simulink model "CyberSuspension_MultiBlock"  (R2024b)
settings: Solver=ode4  StartTime=0.0  StopTime=10  FixedStep=0.001  RelTol=1e-3
settings Model: Creator=sange  LastModifiedBy=sange
settings DataIOCC: SaveOutput=off

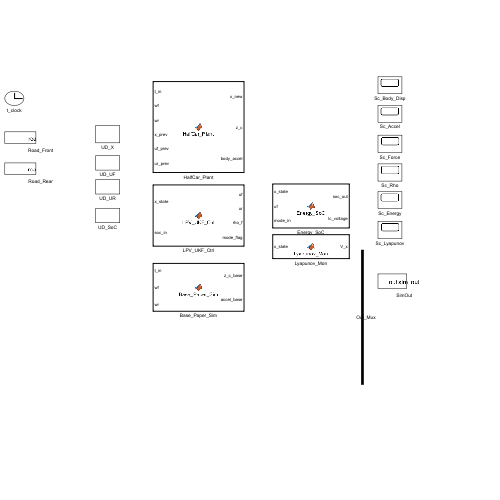
[thumbnail: Simulink's stored preview of the top-level diagram]
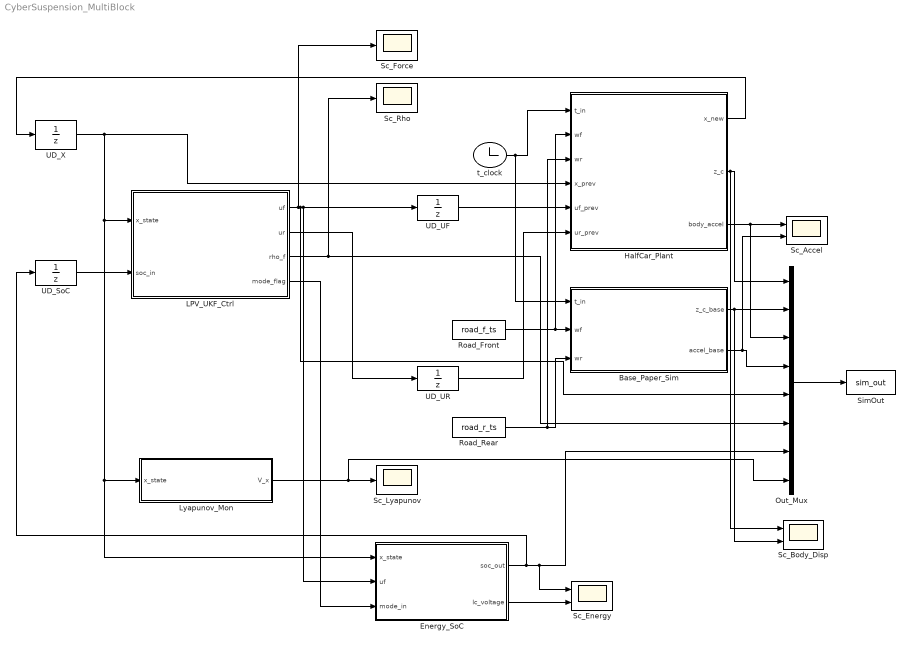
== system CyberSuspension_MultiBlock ==
  Base_Paper_Sim : MATLAB Function  TreatAsAtomicUnit=on
  Energy_SoC : MATLAB Function  TreatAsAtomicUnit=on
  HalfCar_Plant : MATLAB Function  TreatAsAtomicUnit=on
  LPV_UKF_Ctrl : MATLAB Function  TreatAsAtomicUnit=on
  Lyapunov_Mon : MATLAB Function  TreatAsAtomicUnit=on
  Out_Mux : Mux  Inputs=8
  Road_Front : FromWorkspace  VariableName=road_f_ts
  Road_Rear : FromWorkspace  VariableName=road_r_ts
  Sc_Accel : Scope  NumInputPorts=2
  Sc_Body_Disp : Scope  NumInputPorts=2
  Sc_Energy : Scope  NumInputPorts=2
  Sc_Force : Scope
  Sc_Lyapunov : Scope
  Sc_Rho : Scope
  SimOut : ToWorkspace  VariableName=sim_out  SaveFormat=Structure With Time  SampleTime=-1
  UD_SoC : UnitDelay  InitialCondition=0.5  SampleTime=0.001  HasFrameUpgradeWarning=on
  UD_UF : UnitDelay  SampleTime=0.001  HasFrameUpgradeWarning=on
  UD_UR : UnitDelay  SampleTime=0.001  HasFrameUpgradeWarning=on
  UD_X : UnitDelay  InitialCondition=zeros(8,1)  SampleTime=0.001  HasFrameUpgradeWarning=on
  t_clock : Clock
  wires:
  Lyapunov_Mon/1(V_x) -> Sc_Lyapunov/1, Out_Mux/8
  UD_SoC/1 -> LPV_UKF_Ctrl/2(soc_in)
  UD_X/1 -> Energy_SoC/1(x_state), Lyapunov_Mon/1(x_state), LPV_UKF_Ctrl/1(x_state), HalfCar_Plant/4(x_prev)
  LPV_UKF_Ctrl/4(mode_flag) -> Energy_SoC/3(mode_in)
  LPV_UKF_Ctrl/3(rho_f) -> Sc_Rho/1, Out_Mux/6
  Energy_SoC/2(lc_voltage) -> Sc_Energy/2
  LPV_UKF_Ctrl/1(uf) -> UD_UF/1, Energy_SoC/2(uf), Out_Mux/5, Sc_Force/1
  t_clock/1 -> Base_Paper_Sim/1(t_in), HalfCar_Plant/1(t_in)
  LPV_UKF_Ctrl/2(ur) -> UD_UR/1
  UD_UF/1 -> HalfCar_Plant/5(uf_prev)
  Road_Rear/1 -> HalfCar_Plant/3(wr), Base_Paper_Sim/3(wr)
  Road_Front/1 -> HalfCar_Plant/2(wf), Base_Paper_Sim/2(wf)
  UD_UR/1 -> HalfCar_Plant/6(ur_prev)
  Energy_SoC/1(soc_out) -> Out_Mux/7, Sc_Energy/1, UD_SoC/1
  HalfCar_Plant/2(z_c) -> Sc_Body_Disp/1, Out_Mux/1
  HalfCar_Plant/1(x_new) -> UD_X/1
  HalfCar_Plant/3(body_accel) -> Sc_Accel/1, Out_Mux/3
  Base_Paper_Sim/1(z_c_base) -> Sc_Body_Disp/2, Out_Mux/2
  Base_Paper_Sim/2(accel_base) -> Sc_Accel/2, Out_Mux/4
  Out_Mux/1 -> SimOut/1

== matlab function CyberSuspension_MultiBlock/LPV_UKF_Ctrl ==
  data: x_state input; uf output; soc_in input; ur output; rho_f output; mode_flag output
function [uf, ur, rho_f, mode_flag] = LPV_UKF_Ctrl(x_state, soc_in)
% LPV-Adaptive H-inf Controller with UKF Road Estimator + TD3 Heuristic
% Block 2 in the signal chain. Uses x_state from Unit Delay (1ms behind plant).
persistent rho_f_p rdot_filt mets_last mets_first

a=1.10; b=1.50;
C_e=1500; u_max=6000; sig_m=0.10;
w_max=0.05; ema_a=0.05; dt=0.001;
Ks  = [2591.260282 2545.019204 -4409.593492 -22.6009354];
Kr  = [1339.079606 6792.410633 -15288.11257 39.41237591];
Krd = [0 500 0 0];

% Initialise persistent variables (auto-reset at start of each sim run)
if isempty(rho_f_p)
    rho_f_p=0; rdot_filt=0; mets_last=zeros(8,1); mets_first=true;
end

% ---- Step A: METS Network Filter ----
if mets_first
    net=x_state; mets_last=x_state; mets_first=false;
else
    em=x_state-mets_last;
    nx=sqrt(sum(x_state.^2)); ne=sqrt(sum(em.^2));
    if ne>sig_m*nx; mets_last=x_state; net=x_state;
    else;           net=mets_last; end
end

% ---- Step B: UKF Road Estimator (algebraic proxy) ----
rho_f     = min(1, max(0, abs(x_state(1)-a*x_state(2)-x_state(3)) / w_max));
rdot_filt = ema_a*((rho_f-rho_f_p)/dt) + (1-ema_a)*rdot_filt;
rho_dot   = rdot_filt;  rho_f_p = rho_f;

% ---- Step C: TD3 Heuristic Energy Agent ----
if rho_f>0.7 || rho_dot>0.5
    if soc_in<0.02; mf=1; else; mf=0; end   % COMFORT if SoC critical
elseif rho_f>0.3
    if soc_in<0.25; mf=1; else; mf=0; end
else
    mf=1;  % Smooth road — harvest energy (ECO)
end

% ---- Step D: LPV Controller — Polytopic Gain Scheduling ----
zsf=net(1)-a*net(2); zsfd=net(5)-a*net(6); qcf=[zsf-net(3);zsfd;0;net(7)];
zsr=net(1)+b*net(2); zsrd=net(5)+b*net(6); qcr=[zsr-net(4);zsrd;0;net(8)];
ffl = 0.2*u_max;
if mf==1  % ECO: passive regenerative damping
    uf=-C_e*qcf(2);  ur=-C_e*qcr(2);
else       % COMFORT: blended LPV H-inf + feedforward
    Kf = (1-rho_f)*Ks + rho_f*Kr;   % Polytopic interpolation
    uf = (-Kf*qcf) + max(-ffl, min(ffl, -Krd*max(0,rho_dot)*qcf));
    ur = (-Kf*qcr) + max(-ffl, min(ffl, -Krd*max(0,rho_dot)*qcr));
end
uf=max(-u_max,min(u_max,uf));  ur=max(-u_max,min(u_max,ur));
mode_flag = double(mf);
end

== matlab function CyberSuspension_MultiBlock/HalfCar_Plant ==
  data: t_in input; x_new output; wf input; wr input; x_prev input; uf_prev input; ur_prev input; z_c output; body_accel output
function [x_new, z_c, body_accel] = HalfCar_Plant(t_in, wf, wr, x_prev, uf_prev, ur_prev)
% 4-DOF Half-Car Plant with RK4 Integration
% State: [z_c, theta, z_uf, z_ur, z_c_dot, theta_dot, z_uf_dot, z_ur_dot]
% State passed explicitly — no persistent variables needed here.

ms=730.0;  I_phi=1222.0;  a=1.10;  b=1.50;
mu_f=45.0; mu_r=45.0;
ks_f=18000; ks_r=22000; cs_f=1200; cs_r=1200;
kt_f=190000; kt_r=190000;
k_em=15.0; i_d=20.0; p_pole=8; whr=0.30; v_ms=20.00;
smax=0.0800; u_max=6000; k_bs=1.00e+07;
dt = 0.001;

% Runge-Kutta 4 integration (fixed-step, dt=1ms)
k1=hc_ode(t_in,      x_prev,         uf_prev,ur_prev,wf,wr,ms,I_phi,a,b,mu_f,mu_r,ks_f,ks_r,cs_f,cs_r,kt_f,kt_r,k_em,i_d,p_pole,whr,v_ms,smax,k_bs);
k2=hc_ode(t_in+dt/2, x_prev+k1*dt/2, uf_prev,ur_prev,wf,wr,ms,I_phi,a,b,mu_f,mu_r,ks_f,ks_r,cs_f,cs_r,kt_f,kt_r,k_em,i_d,p_pole,whr,v_ms,smax,k_bs);
k3=hc_ode(t_in+dt/2, x_prev+k2*dt/2, uf_prev,ur_prev,wf,wr,ms,I_phi,a,b,mu_f,mu_r,ks_f,ks_r,cs_f,cs_r,kt_f,kt_r,k_em,i_d,p_pole,whr,v_ms,smax,k_bs);
k4=hc_ode(t_in+dt,   x_prev+k3*dt,   uf_prev,ur_prev,wf,wr,ms,I_phi,a,b,mu_f,mu_r,ks_f,ks_r,cs_f,cs_r,kt_f,kt_r,k_em,i_d,p_pole,whr,v_ms,smax,k_bs);
x_new      = x_prev + (dt/6)*(k1 + 2*k2 + 2*k3 + k4);
z_c        = x_new(1);
body_accel = k1(5);
end

function dx = hc_ode(t,x,uf,ur,wf,wr,ms,Ip,a,b,muf,mur,ksf,ksr,csf,csr,ktf,ktr,kem,id,pp,whr,vms,sm,kbs)
    z_c=x(1);th=x(2);zuf=x(3);zur=x(4);zcd=x(5);thd=x(6);zufd=x(7);zurd=x(8);
    zsf=z_c-a*th; zsr=z_c+b*th; zsfd=zcd-a*thd; zsrd=zcd+b*thd;
    dsf=zsf-zuf; dsr=zsr-zur; dtf=zuf-wf; dtr=zur-wr;
    vrf=zsfd-zufd; vrr=zsrd-zurd;
    if dsf> sm; fbf=kbs*(dsf-sm)^3; elseif dsf<-sm; fbf=kbs*(dsf+sm)^3; else; fbf=0; end
    if dsr> sm; fbr=kbs*(dsr-sm)^3; elseif dsr<-sm; fbr=kbs*(dsr+sm)^3; else; fbr=0; end
    fiwm = kem*id*sin(pp*(vms/whr)*t);
    Fsf=ksf*dsf+csf*vrf+fbf-uf; Fsr=ksr*dsr+csr*vrr+fbr-ur;
    dx=[zcd;thd;zufd;zurd; -(Fsf+Fsr)/ms; (a*Fsf-b*Fsr)/Ip; (Fsf-ktf*dtf+fiwm)/muf; (Fsr-ktr*dtr+fiwm)/mur];
end

== matlab function CyberSuspension_MultiBlock/Energy_SoC ==
  data: x_state input; soc_out output; uf input; mode_in input; lc_voltage output
function [soc_out, lc_voltage] = Energy_SoC(x_state, uf, mode_in)
% LC Filter Power Electronics + Regenerative Energy Harvesting
% Tracks battery State-of-Charge and LC filter capacitor voltage.
persistent bat_soc lc_il lc_vc

a=1.10; K_v=50.0; eta_r=0.65; eta_act=0.85;
Lf=0.0100; Cf=0.004700; Rl=10.0; cap_j=50000; dt=0.001;
N_t=10.0; % Lightweight Transformer/Boost step-up ratio

if isempty(bat_soc); bat_soc=0.5; lc_il=0; lc_vc=0; end

% Relative suspension velocity (front corner)
vrf = (x_state(5) - a*x_state(6)) - x_state(7);

if mode_in == 1  % ECO mode: harvest energy via back-EMF
    v_rect = abs(K_v * vrf) * N_t; % Voltage is boosted by transformer
    di_L   = (v_rect - lc_vc) / Lf;
    dv_C   = (lc_il - lc_vc/Rl) / Cf;
    lc_il  = min(max(lc_il + di_L*dt, 0), 100);  % Clamped
    lc_vc  = min(max(lc_vc + dv_C*dt, 0), 500);
    bat_soc = min(1.0, bat_soc + (lc_vc^2/Rl)*eta_r*dt / cap_j);
else             % COMFORT mode: active actuator consumes battery
    bat_soc = max(0.0, bat_soc - abs(uf*vrf)/eta_act*dt / cap_j);
    lc_il = lc_il*0.99;  lc_vc = lc_vc*0.99;  % LC filter decays
end

soc_out    = bat_soc;
lc_voltage = lc_vc;
end

== matlab function CyberSuspension_MultiBlock/Lyapunov_Mon ==
  data: x_state input; V_x output
function V_x = Lyapunov_Mon(x_state)
% Lyapunov Stability Monitor  V(x) = x_qc' * P * x_qc
% V(x) must be positive and decreasing for Lyapunov stability.
% P is the solution to CARE with Q=diag([1e5,1e4,1e4,1e2]), R=1e-3.
a  = 1.10;
Pl = [55514.66518 1292.584418 51939.7711 21.505047;1292.584418 1223.579227 -1867.584611 16.21273818;51939.7711 -1867.584611 68939.36182 -1.11842938;21.505047 16.21273818 -1.11842938 2.749362062];

% Map half-car state to front quarter-car state vector
xq  = [x_state(1)-a*x_state(2)-x_state(3); ...
        x_state(5)-a*x_state(6); 0; x_state(7)];
V_x = xq' * Pl * xq;
end

== matlab function CyberSuspension_MultiBlock/Base_Paper_Sim ==
  data: t_in input; z_c_base output; wf input; wr input; accel_base output
function [z_c_base, accel_base] = Base_Paper_Sim(t_in, wf, wr)
% Fixed H-infinity Base Paper Controller (self-contained with persistent state)
% Used as a performance baseline — no gain scheduling, no energy harvesting.
persistent st_base

ms=730.0; I_phi=1222.0; a=1.10; b=1.50;
mu_f=45.0; mu_r=45.0;
ks_f=18000; ks_r=22000; cs_f=1200; cs_r=1200;
kt_f=190000; kt_r=190000;
k_em=15.0; i_d=20.0; p_pole=8; whr=0.30; v_ms=20.00;
smax=0.0800; u_max=6000; k_bs=1.00e+07; dt=0.001;
Kbf = [-12000 5500 8000 0 -3500 1800 2200 0];
Kbr = [-12000 -5500 0 8000 -3500 -1800 0 2200];

if isempty(st_base); st_base=zeros(8,1); end

uf_b = max(-u_max, min(u_max, -Kbf * st_base));
ur_b = max(-u_max, min(u_max, -Kbr * st_base));
[st_base, dx_b] = rk4_b(t_in,st_base,uf_b,ur_b,wf,wr,ms,I_phi,a,b,mu_f,mu_r,ks_f,ks_r,cs_f,cs_r,kt_f,kt_r,k_em,i_d,p_pole,whr,v_ms,smax,k_bs,dt);
z_c_base   = st_base(1);
accel_base = dx_b(5);
end

function [ns,k1]=rk4_b(t,x,uf,ur,wf,wr,ms,Ip,a,b,muf,mur,ksf,ksr,csf,csr,ktf,ktr,kem,id,pp,whr,vms,sm,kbs,dt)
    k1=ode_b(t,      x,         uf,ur,wf,wr,ms,Ip,a,b,muf,mur,ksf,ksr,csf,csr,ktf,ktr,kem,id,pp,whr,vms,sm,kbs);
    k2=ode_b(t+dt/2, x+k1*dt/2, uf,ur,wf,wr,ms,Ip,a,b,muf,mur,ksf,ksr,csf,csr,ktf,ktr,kem,id,pp,whr,vms,sm,kbs);
    k3=ode_b(t+dt/2, x+k2*dt/2, uf,ur,wf,wr,ms,Ip,a,b,muf,mur,ksf,ksr,csf,csr,ktf,ktr,kem,id,pp,whr,vms,sm,kbs);
    k4=ode_b(t+dt,   x+k3*dt,   uf,ur,wf,wr,ms,Ip,a,b,muf,mur,ksf,ksr,csf,csr,ktf,ktr,kem,id,pp,whr,vms,sm,kbs);
    ns=x+(dt/6)*(k1+2*k2+2*k3+k4);
end

function dx=ode_b(t,x,uf,ur,wf,wr,ms,Ip,a,b,muf,mur,ksf,ksr,csf,csr,ktf,ktr,kem,id,pp,whr,vms,sm,kbs)
    z_c=x(1);th=x(2);zuf=x(3);zur=x(4);zcd=x(5);thd=x(6);zufd=x(7);zurd=x(8);
    zsf=z_c-a*th;zsr=z_c+b*th;zsfd=zcd-a*thd;zsrd=zcd+b*thd;
    dsf=zsf-zuf;dsr=zsr-zur;dtf=zuf-wf;dtr=zur-wr;vrf=zsfd-zufd;vrr=zsrd-zurd;
    if dsf>sm;fbf=kbs*(dsf-sm)^3;elseif dsf<-sm;fbf=kbs*(dsf+sm)^3;else;fbf=0;end
    if dsr>sm;fbr=kbs*(dsr-sm)^3;elseif dsr<-sm;fbr=kbs*(dsr+sm)^3;else;fbr=0;end
    fiwm=kem*id*sin(pp*(vms/whr)*t);
    Fsf=ksf*dsf+csf*vrf+fbf-uf;Fsr=ksr*dsr+csr*vrr+fbr-ur;
    dx=[zcd;thd;zufd;zurd;-(Fsf+Fsr)/ms;(a*Fsf-b*Fsr)/Ip;(Fsf-ktf*dtf+fiwm)/muf;(Fsr-ktr*dtr+fiwm)/mur];
end
